simulink model "SPWM_jisuan_simscape"  (R2026a)
settings: Solver=ode23t  StartTime=1  StopTime=2
undefined symbols (not defined in the file): Down, PermanentMagnetSynchrono_class, Up
libraries: fl_lib x12, nesl_utility x10, ee_lib x4, eePwmGenerator x3, eeTransforms x2, elec_conv_HighZElecRef x1
settings Model: Creator=刘炳宏  LastModifiedBy=mushen
settings DebuggingCC: SaveWithParameterizedLinksMsg=none
settings SimscapeCC: SimscapeLogType=none  SimscapeLogDataHistory=5000.0

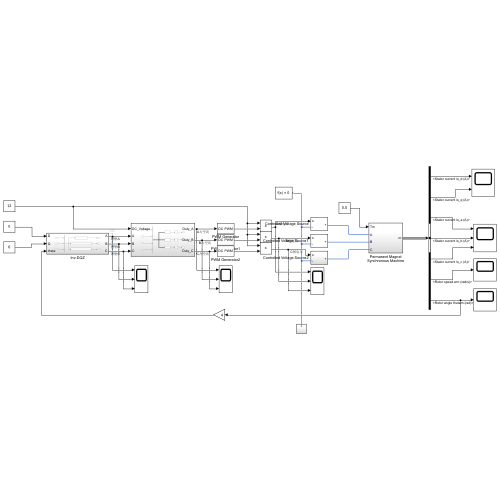
[thumbnail: Simulink's stored preview of the top-level diagram]
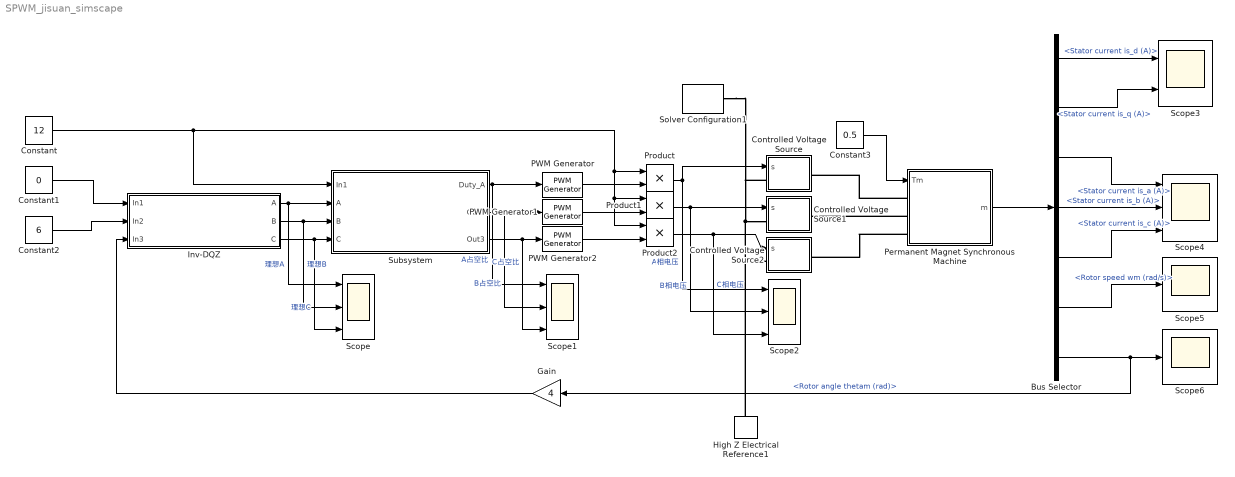
== system SPWM_jisuan_simscape ==
  Bus Selector : BusSelector  OutputSignals=Stator current is_d (A),Stator current is_q (A),Stator current is_a (A),Stator current is_b (A),Stator current is_c (A),Rotor speed wm (rad/s),Rotor angle thetam (rad)
  Constant : Constant  Value=12
  Constant1 : Constant  Value=0
  Constant2 : Constant  Value=6
  Constant3 : Constant  Value=0.5
  Controlled Voltage Source : Subsystem
      settings: OpenFcn=elec.conv.unmask(gcb);
  Controlled Voltage Source1 : Subsystem
      settings: OpenFcn=elec.conv.unmask(gcb);
  Controlled Voltage Source2 : Subsystem
  Gain : Gain  Gain=4
  High Z Electrical Reference1 : elec_conv_HighZElecRef/High Z Electrical Reference  SystemSampleTime=-1  VariantActivationTime=update diagram  EmptyChoice=off  PassThrough=off  PassThroughVariantControl=(default)  EmptyChoiceVariantControl=(default)  AllowFlexibleInterface=on  Latency=0  AutoFrameSizeCalculation=off
  Inv-DQZ : Subsystem
  PWM Generator : eePwmGenerator/PWM Generator  CarrCount=Up-Down  Tper=0.0001  Tdelay=0  Ts=5e-6
  PWM Generator1 : eePwmGenerator/PWM Generator  CarrCount=Up-Down  Tper=0.0001  Tdelay=0  Ts=5e-6
  PWM Generator2 : eePwmGenerator/PWM Generator  CarrCount=Up-Down  Tper=0.0001  Tdelay=0  Ts=5e-6
  Permanent Magnet Synchronous Machine : Subsystem
  Product : Product
  Product1 : Product
  Product2 : Product
  Scope{,1..2,4} (4 alike) : Scope  NumInputPorts=3
      Scope settings: ActiveDisplayYMinimum=-25  ActiveDisplayYMaximum=25
      Scope1 settings: ActiveDisplayYMinimum=-0.12499999999999997  ActiveDisplayYMaximum=1.125
      Scope2 settings: ActiveDisplayYMinimum=-1.5  ActiveDisplayYMaximum=13.5  DataLoggingVariableName=ScopeData2
      Scope4 settings: ActiveDisplayYMinimum=-3.47944  ActiveDisplayYMaximum=3.68146  DataLoggingVariableName=ScopeData4
  Scope3 : Scope  NumInputPorts=2
      settings: ActiveDisplayYMinimum=-3.3984401436548075  ActiveDisplayYMaximum=6.0425246459307287  DataLoggingVariableName=ScopeData3
  Scope5 : Scope
      settings: ActiveDisplayYMinimum=-5.36888  ActiveDisplayYMaximum=42.81454  DataLoggingVariableName=ScopeData5
  Scope6 : Scope
      settings: ActiveDisplayYMinimum=0.00745  ActiveDisplayYMaximum=0.02745  DataLoggingVariableName=ScopeData6
  Solver Configuration1 : nesl_utility/Solver Configuration  PhysicalDomain=network_engine_domain  SubClassName=solver  LeftPortType=input  RightPortType=generic  Tones=[]  Harmonics=[]  SimulateNoise=off  Profile=off  UseLocalSampling=off  EnableSwitchedLinearOptims=on  FrequencyDomain=off  UseCCode=off  RelTol=0.001  AbsTol=0.001  MinStep=1e-09  ToWorkspace=off  RevertToSquareIcSolve=off  NumHomotopyIterations=100  PhasorMode=off  PhasorModeNumHarmonics=1  ConsistencySolver=NEWTON_XTOL_AFTER_FTOL  CanonicalOrdering=CANONICAL  OptimizeIntermediates=OPTIMIZED  IndexReductionMethod=DerivativeReplacement  DoDC=off  ResidualTolerance=1e-09  ConsistencyTolSource=GLOBAL  ConsistencyAbsTol=0.001  ConsistencyRelTol=0.001  ConsistencyTolFactor=0.001  UseLocalSolver=off  LocalSolverChoice=NE_BACKWARD_EULER_ADVANCER  ResolveIndetEquations=on  FunctionEvalNumThread=1  LocalSolverSampleTime=0.001  DoFixedCost=off  MaxNonlinIter=3  MaxModeIter=2  ComputeImpulses=off  ImpulseIterations=2  LinearAlgebra=auto  LinearAlgebraNumThread=0  EquationFormulation=NE_TIME_EF  DelaysMemoryBudget=1024  AutomaticFiltering=on  FilteringTimeConstant=0.001  PartitionStorageMethod=AS_NEEDED  PartitionMemoryBudget=1024  PartitionMethod=ROBUST  MultibodyUseLocalSolver=off  MultibodyLocalSolverChoice=ODE1  MultibodyLocalSolverSampleTime=0.001
  Subsystem : Subsystem
  wires:
  Inv-DQZ/2(B) -> Scope/2, Subsystem/3(B)  "理想B"
  Inv-DQZ/3(C) -> Scope/3, Subsystem/4(C)  "理想C"
  Inv-DQZ/1(A) -> Scope/1, Subsystem/2(A)  "理想A"
  Subsystem/1(Duty_A) -> PWM Generator/1, Scope1/1  "A占空比"
  Subsystem/2(Out2) -> PWM Generator1/1, Scope1/2  "B占空比"
  Subsystem/3(Out3) -> PWM Generator2/1, Scope1/3  "C占空比"
  PWM Generator/1 -> Product/2
  PWM Generator1/1 -> Product1/2
  PWM Generator2/1 -> Product2/2
  Constant/1 -> Product2/1, Product1/1, Product/1, Subsystem/1(In1)
  Constant1/1 -> Inv-DQZ/1(In1)
  Constant2/1 -> Inv-DQZ/2(In2)
  Constant3/1 -> Permanent Magnet Synchronous Machine/1(Tm)
  Product/1 -> Scope2/1, Controlled Voltage Source/1(s)  "A相电压"
  Product1/1 -> Scope2/2, Controlled Voltage Source1/1(s)  "B相电压"
  Product2/1 -> Scope2/3, Controlled Voltage Source2/1(s)  "C相电压"
  Permanent Magnet Synchronous Machine/1(m) -> Bus Selector/1
  Bus Selector/1 -> Scope3/1  "<Stator current is_d (A)>"
  Bus Selector/2 -> Scope3/2  "<Stator current is_q (A)>"
  Bus Selector/4 -> Scope4/2  "<Stator current is_b (A)>"
  Bus Selector/3 -> Scope4/1  "<Stator current is_a (A)>"
  Bus Selector/5 -> Scope4/3  "<Stator current is_c (A)>"
  Bus Selector/6 -> Scope5/1  "<Rotor speed wm (rad/s)>"
  Bus Selector/7 -> Gain/1, Scope6/1  "<Rotor angle thetam (rad)>"
  Gain/1 -> Inv-DQZ/3(In3)
  connections:
  Permanent Magnet Synchronous Machine/LConn2 -- Controlled Voltage Source1/RConn1
  Permanent Magnet Synchronous Machine/LConn3 -- Controlled Voltage Source2/RConn1
  Permanent Magnet Synchronous Machine/LConn1 -- Controlled Voltage Source/RConn1
  Controlled Voltage Source/LConn1 -- Solver Configuration1/RConn1 -- Controlled Voltage Source1/LConn1 -- Controlled Voltage Source2/LConn1 -- High Z Electrical Reference1/LConn1

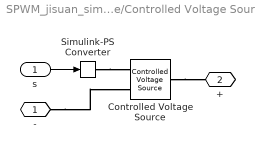
== system SPWM_jisuan_simscape/Controlled Voltage Source ==
  s : Inport
  Controlled Voltage Source : fl_lib/Electrical/Electrical Sources/Controlled Voltage Source
  Simulink-PS Converter : nesl_utility/Simulink-PS Converter  PhysicalDomain=network_engine_domain  SubClassName=ps_input  LeftPortType=input  RightPortType=output  PseudoPeriodic=off  Frequencies=[]  NoiseDistribution=none  NoiseParameters=[]  Unit=1  AffineConversion=off  FilteringAndDerivatives=provide  SimscapeFilterOrder=1  InputFilterTimeConstant=0.001  UdotUserProvided=0
  - : PMIOPort  Side=Left
  + : PMIOPort  Port=2  Side=Right
  wires:
  s/1 -> Simulink-PS Converter/1
  connections:
  -/RConn1 -- Controlled Voltage Source/RConn2
  Simulink-PS Converter/RConn1 -- Controlled Voltage Source/RConn1
  Controlled Voltage Source/LConn1 -- +/RConn1

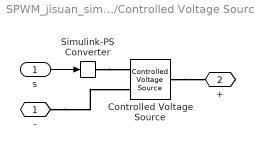
== system SPWM_jisuan_simscape/Controlled Voltage Source1 ==
  s : Inport
  Controlled Voltage Source : fl_lib/Electrical/Electrical Sources/Controlled Voltage Source
  Simulink-PS Converter : nesl_utility/Simulink-PS Converter  PhysicalDomain=network_engine_domain  SubClassName=ps_input  LeftPortType=input  RightPortType=output  PseudoPeriodic=off  Frequencies=[]  NoiseDistribution=none  NoiseParameters=[]  Unit=1  AffineConversion=off  FilteringAndDerivatives=provide  SimscapeFilterOrder=1  InputFilterTimeConstant=0.001  UdotUserProvided=0
  - : PMIOPort  Side=Left
  + : PMIOPort  Port=2  Side=Right
  wires:
  s/1 -> Simulink-PS Converter/1
  connections:
  -/RConn1 -- Controlled Voltage Source/RConn2
  Simulink-PS Converter/RConn1 -- Controlled Voltage Source/RConn1
  Controlled Voltage Source/LConn1 -- +/RConn1

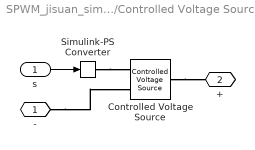
== system SPWM_jisuan_simscape/Controlled Voltage Source2 ==
  s : Inport
  Controlled Voltage Source : fl_lib/Electrical/Electrical Sources/Controlled Voltage Source
  Simulink-PS Converter : nesl_utility/Simulink-PS Converter  PhysicalDomain=network_engine_domain  SubClassName=ps_input  LeftPortType=input  RightPortType=output  PseudoPeriodic=off  Frequencies=[]  NoiseDistribution=none  NoiseParameters=[]  Unit=1  AffineConversion=off  FilteringAndDerivatives=provide  SimscapeFilterOrder=1  InputFilterTimeConstant=0.001  UdotUserProvided=0
  - : PMIOPort  Side=Left
  + : PMIOPort  Port=2  Side=Right
  wires:
  s/1 -> Simulink-PS Converter/1
  connections:
  -/RConn1 -- Controlled Voltage Source/RConn2
  Simulink-PS Converter/RConn1 -- Controlled Voltage Source/RConn1
  Controlled Voltage Source/LConn1 -- +/RConn1

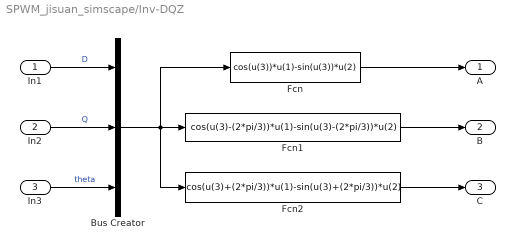
== system SPWM_jisuan_simscape/Inv-DQZ ==
  In1 : Inport
  In2 : Inport  Port=2
  In3 : Inport  Port=3
  Bus Creator : BusCreator  Inputs=3
  Fcn : Fcn  Expr=cos(u(3))*u(1)-sin(u(3))*u(2)
  Fcn1 : Fcn  Expr=cos(u(3)-(2*pi/3))*u(1)-sin(u(3)-(2*pi/3))*u(2)
  Fcn2 : Fcn  Expr=cos(u(3)+(2*pi/3))*u(1)-sin(u(3)+(2*pi/3))*u(2)
  A : Outport
  B : Outport  Port=2
  C : Outport  Port=3
  wires:
  In3/1 -> Bus Creator/3  "theta"
  In2/1 -> Bus Creator/2  "Q"
  In1/1 -> Bus Creator/1  "D"
  Bus Creator/1 -> Fcn/1, Fcn1/1, Fcn2/1
  Fcn/1 -> A/1
  Fcn1/1 -> B/1
  Fcn2/1 -> C/1

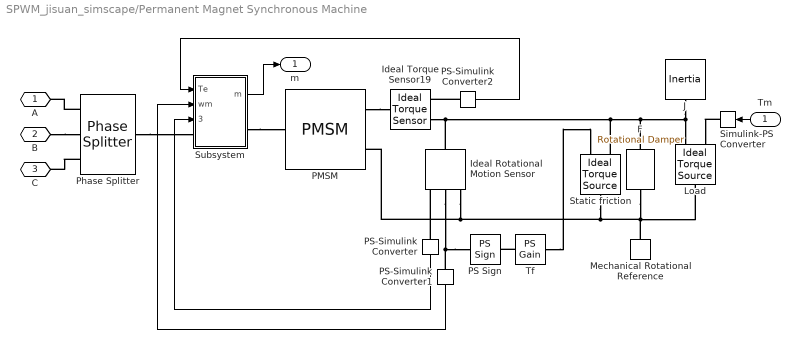
== system SPWM_jisuan_simscape/Permanent Magnet Synchronous Machine ==
  Tm : Inport
  F : fl_lib/Mechanical/Rotational Elements/Rotational Damper  D=0.0003505 N*m/(rad/s)  w_specify=on  w_priority=High  w=0 rad/s  w_nominal_specify=off  w_nominal_value=1  w_nominal_unit=rad/s  t_specify=off  t_priority=None  t=0 N*m  t_nominal_specify=off  t_nominal_value=1  t_nominal_unit=N*m
  Ideal Rotational Motion Sensor : fl_lib/Mechanical/Mechanical Sensors/Ideal Rotational Motion Sensor  reference=foundation.enum.MeasurementReference.difference  acceleration_port=false  velocity_port=true  position_port=true  wrap_angle=simscape.enum.onoff.off  offset=1 deg
  Ideal Torque Sensor19 : fl_lib/Mechanical/Mechanical Sensors/Ideal Torque Sensor
  J : fl_lib/Mechanical/Rotational Elements/Inertia  inertia=0.00062 kg*m^2  num_ports=foundation.enum.numPorts2.one  w_specify=on  w_priority=High  w=0 rad/s  w_nominal_specify=off  w_nominal_value=1  w_nominal_unit=rad/s  t_specify=off  t_priority=None  t=0 N*m  t_nominal_specify=off  t_nominal_value=1  t_nominal_unit=N*m
  Load : fl_lib/Mechanical/Mechanical Sources/Ideal Torque Source
  Mechanical Rotational Reference : fl_lib/Mechanical/Rotational Elements/Mechanical Rotational Reference
  PMSM : ee_lib/Electromechanical/Permanent Magnet/PMSM  port_option=ee.enum.threePhasePort.composite  winding_type=ee.enum.statorconnection.wye  machine_param=ee.enum.pmsm.parameterization.constant  nPolePairs=4  pmflux_param=1  pm_flux_linkage=PermanentMagnetSynchrono_class('Torque Tm',[0.00062 0.0003505 4 0],4,'Flux linkage established by magnets (V.s)',0.074147,53.7951,0.44488,'Aligned with phase A axis (original Park)',[0 1 0 0],'Sinusoidal',120,'3',[0 0 0 0 0 0]).objParamMappingDerived.NewDerivedParam.pm_flux_linkage Wb  torque_constant=0.18 N*m/A  back_emf_constant=0.18 V/(rad/s)  stator_param=1  Ld=0.0085 H  Lq=0.0085 H  idVec=[-200, 0, 200] A  iqVec=[-200, 0, 200] A  LdMatrix=0.0002 * ones(3, 3) H  LqMatrix=0.0002 * ones(3, 3) H  PmMatrix=0.1 * ones(3, 3) Wb  ktMatrix=0.18 * ones(3, 3) N*m/A  keMatrix=0.18 * ones(3, 3) V/(rad/s)  L0=1e-09 H  Ls=0.0002 H  Lm=-0.00002 H  Ms=0.00002 H  Rs=0.18 Ohm  zero_sequence=0  axes_param=2  loss_param=ee.enum.ironloss.none  losses_oc=[0, 0, 0] W  losses_sc=[0, 0, 0] W  f_losses=60 Hz  Isc_losses=95 A  J=0 kg*m^2  lam=0 N*m/(rad/s)  i_d_specify=on  i_d_priority=High  i_d=PermanentMagnetSynchrono_class('Torque Tm',[0.00062 0.0003505 4 0],4,'Flux linkage established by magnets (V.s)',0.074147,53.7951,0.44488,'Aligned with phase A axis (original Park)',[0 1 0 0],'Sinusoidal',120,'3',[0 0 0 0 0 0]).objParamMappingDerived.NewDerivedParam.i_d A  i_d_nominal_specify=off  i_d_nominal_value=1  i_d_nominal_unit=A  i_q_specify=on  i_q_priority=High  i_q=PermanentMagnetSynchrono_class('Torque Tm',[0.00062 0.0003505 4 0],4,'Flux linkage established by magnets (V.s)',0.074147,53.7951,0.44488,'Aligned with phase A axis (original Park)',[0 1 0 0],'Sinusoidal',120,'3',[0 0 0 0 0 0]).objParamMappingDerived.NewDerivedParam.i_q A  i_q_nominal_specify=off  i_q_nominal_value=1  i_q_nominal_unit=A  torque_specify=off  torque_priority=None  torque=0 N*m  torque_nominal_specify=off  torque_nominal_value=1  torque_nominal_unit=N*m  angular_velocity_specify=on  angular_velocity_priority=High  angular_velocity=0 rad/s  angular_velocity_nominal_specify=off  angular_velocity_nominal_value=1  angular_velocity_nominal_unit=rpm  angular_position_specify=on  angular_position_priority=High  angular_position=1 deg  angular_position_nominal_specify=off  angular_position_nominal_value=1  angular_position_nominal_unit=deg  alpha=3.93e-3 1/K  alpha_flux=-0.001 1/K  Tmeas=298.15 K  stator_thermal_mass=100 J/K  rotor_thermal_mass=200 J/K  Rm_percent_rotor=90  Rd_percent_rotor=30  temperatureA_specify=off  temperatureA_priority=High  temperatureA=25 degC  temperatureA_nominal_specify=off  temperatureA_nominal_value=1  temperatureA_nominal_unit=degC  temperatureB_specify=off  temperatureB_priority=High  temperatureB=25 degC  temperatureB_nominal_specify=off  temperatureB_nominal_value=1  temperatureB_nominal_unit=degC  temperatureC_specify=off  temperatureC_priority=High  temperatureC=25 degC  temperatureC_nominal_specify=off  temperatureC_nominal_value=1  temperatureC_nominal_unit=degC  temperatureR_specify=off  temperatureR_priority=High  temperatureR=25 degC  temperatureR_nominal_specify=off  temperatureR_nominal_value=1  temperatureR_nominal_unit=degC
  PS Sign : fl_lib/Physical Signals/Nonlinear Operators/PS Sign
  PS-Simulink Converter : nesl_utility/PS-Simulink Converter  PhysicalDomain=network_engine_domain  SubClassName=ps_output  LeftPortType=input  RightPortType=output  PseudoPeriodic=off  Frequencies=[]  VectorFormat=1-D array  Unit=1  AffineConversion=off
  PS-Simulink Converter1 : nesl_utility/PS-Simulink Converter  PhysicalDomain=network_engine_domain  SubClassName=ps_output  LeftPortType=input  RightPortType=output  PseudoPeriodic=off  Frequencies=[]  VectorFormat=1-D array  Unit=1  AffineConversion=off
  PS-Simulink Converter2 : nesl_utility/PS-Simulink Converter  PhysicalDomain=network_engine_domain  SubClassName=ps_output  LeftPortType=input  RightPortType=output  PseudoPeriodic=off  Frequencies=[]  VectorFormat=1-D array  Unit=1  AffineConversion=off
  Phase Splitter : ee_lib/Connectors & References/Phase Splitter
  Simulink-PS Converter : nesl_utility/Simulink-PS Converter  PhysicalDomain=network_engine_domain  SubClassName=ps_input  LeftPortType=input  RightPortType=output  PseudoPeriodic=off  Frequencies=[]  NoiseDistribution=none  NoiseParameters=[]  Unit=1  AffineConversion=off  FilteringAndDerivatives=provide  SimscapeFilterOrder=1  InputFilterTimeConstant=0.001  UdotUserProvided=0
  Static friction : fl_lib/Mechanical/Mechanical Sources/Ideal Torque Source
  Subsystem : Subsystem
  Tf : fl_lib/Physical Signals/Functions/PS Gain  gain=PermanentMagnetSynchrono_class('Torque Tm',[0.00062 0.0003505 4 0],4,'Flux linkage established by magnets (V.s)',0.074147,53.7951,0.44488,'Aligned with phase A axis (original Park)',[0 1 0 0],'Sinusoidal',120,'3',[0 0 0 0 0 0]).objParamMappingDerived.NewDerivedParam.Tf
  A : PMIOPort  Side=Left
  B : PMIOPort  Port=2  Side=Left
  C : PMIOPort  Port=3  Side=Left
  m : Outport  VectorParamsAs1DForOutWhenUnconnected=off
  wires:
  PS-Simulink Converter1/1 -> Subsystem/2(wm)
  PS-Simulink Converter/1 -> Subsystem/3(thetam)
  PS-Simulink Converter2/1 -> Subsystem/1(Te)
  Subsystem/1(m) -> m/1
  Tm/1 -> Simulink-PS Converter/1
  connections:
  PS-Simulink Converter2/LConn1 -- Ideal Torque Sensor19/RConn2
  Phase Splitter/LConn1 -- Subsystem/LConn1
  Subsystem/RConn1 -- PMSM/LConn1
  PS-Simulink Converter/LConn1 -- Ideal Rotational Motion Sensor/RConn3
  Tf/RConn1 -- Static friction/RConn1
  PS Sign/LConn1 -- PS-Simulink Converter1/LConn1 -- Ideal Rotational Motion Sensor/RConn2
  Tf/LConn1 -- PS Sign/RConn1
  PMSM/RConn1 -- Ideal Torque Sensor19/LConn1
  Ideal Torque Sensor19/RConn1 -- Static friction/RConn2 -- F/LConn1 -- Load/RConn2 -- J/LConn1 -- Ideal Rotational Motion Sensor/LConn1
  Phase Splitter/RConn3 -- C/RConn1
  Phase Splitter/RConn1 -- A/RConn1
  B/RConn1 -- Phase Splitter/RConn2
  Simulink-PS Converter/RConn1 -- Load/RConn1
  Load/LConn1 -- F/RConn1 -- Static friction/LConn1 -- PMSM/RConn2 -- Ideal Rotational Motion Sensor/RConn1 -- Mechanical Rotational Reference/LConn1

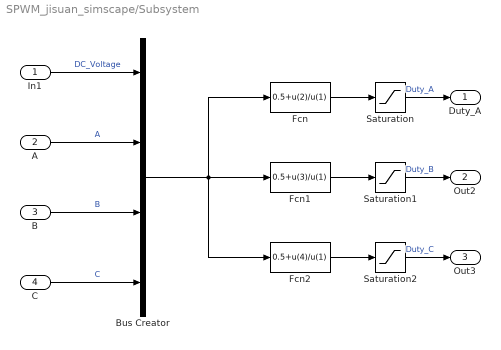
== system SPWM_jisuan_simscape/Subsystem ==
  In1 : Inport
  A : Inport  Port=2
  B : Inport  Port=3
  C : Inport  Port=4
  Bus Creator : BusCreator  Inputs=4
  Fcn : Fcn  Expr=0.5+u(2)/u(1)
  Fcn1 : Fcn  Expr=0.5+u(3)/u(1)
  Fcn2 : Fcn  Expr=0.5+u(4)/u(1)
  Saturation : Saturate  UpperLimit=1  LowerLimit=0
  Saturation1 : Saturate  UpperLimit=1  LowerLimit=0
  Saturation2 : Saturate  UpperLimit=1  LowerLimit=0
  Duty_A : Outport
  Out2 : Outport  Port=2
  Out3 : Outport  Port=3
  wires:
  In1/1 -> Bus Creator/1  "DC_Voltage"
  A/1 -> Bus Creator/2  "A"
  B/1 -> Bus Creator/3  "B"
  C/1 -> Bus Creator/4  "C"
  Fcn/1 -> Saturation/1
  Bus Creator/1 -> Fcn/1, Fcn2/1, Fcn1/1
  Saturation/1 -> Duty_A/1  "Duty_A"
  Saturation1/1 -> Out2/1  "Duty_B"
  Fcn1/1 -> Saturation1/1
  Saturation2/1 -> Out3/1  "Duty_C"
  Fcn2/1 -> Saturation2/1

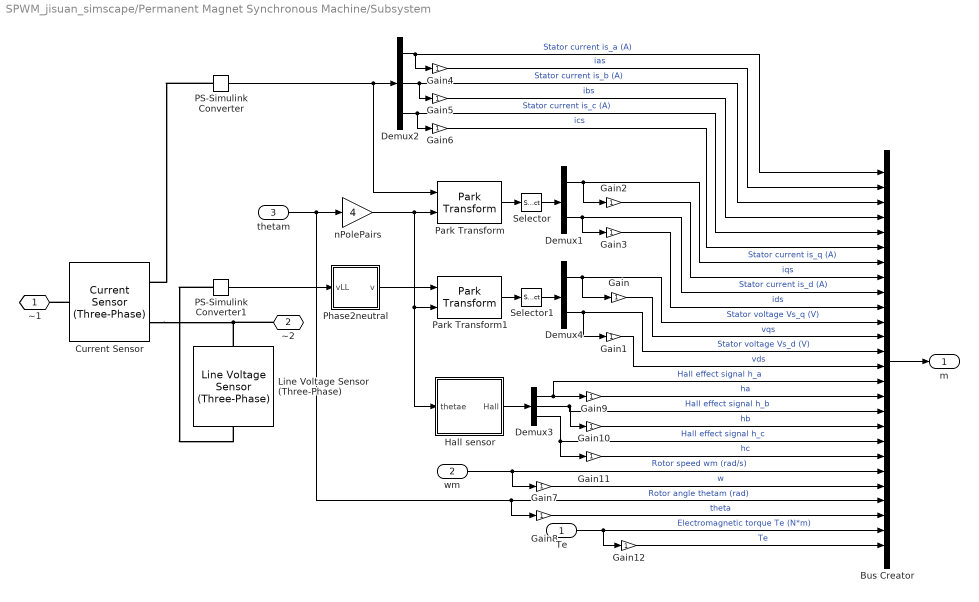
== system SPWM_jisuan_simscape/Permanent Magnet Synchronous Machine/Subsystem ==
  Te : Inport
  wm : Inport  Port=2
  thetam : Inport  Port=3
  Bus Creator : BusCreator  Inputs=26
  Current Sensor : ee_lib/Sensors & Transducers/Current Sensor (Three-Phase)  port_option=ee.enum.threePhasePort.composite
  Demux1 : Demux  Outputs=2
  Demux2 : Demux  Outputs=3
  Demux3 : Demux  Outputs=3
  Demux4 : Demux  Outputs=2
  Gain{,1..12} (13 alike) : Gain
  Hall sensor : Subsystem
  Line Voltage Sensor (Three-Phase) : ee_lib/Sensors & Transducers/Line Voltage Sensor (Three-Phase)  port_option=ee.enum.threePhasePort.composite
  PS-Simulink Converter : nesl_utility/PS-Simulink Converter  PhysicalDomain=network_engine_domain  SubClassName=ps_output  LeftPortType=input  RightPortType=output  PseudoPeriodic=off  Frequencies=[]  VectorFormat=1-D array  Unit=1  AffineConversion=off
  PS-Simulink Converter1 : nesl_utility/PS-Simulink Converter  PhysicalDomain=network_engine_domain  SubClassName=ps_output  LeftPortType=input  RightPortType=output  PseudoPeriodic=off  Frequencies=[]  VectorFormat=1-D array  Unit=1  AffineConversion=off
  Park Transform : eeTransforms/Park Transform  AxisAlignment=D-axis  PowerInvariant=off
  Park Transform1 : eeTransforms/Park Transform  AxisAlignment=D-axis  PowerInvariant=off
  Phase2neutral : Subsystem
  Selector : Selector  InputPortWidth=3  IndexOptions=Index vector (dialog)  Indices=[2 1]  OutputSizes=1
  Selector1 : Selector  InputPortWidth=3  IndexOptions=Index vector (dialog)  Indices=[2 1]  OutputSizes=1
  nPolePairs : Gain  Gain=4
  ~1 : PMIOPort  Side=Left
  ~2 : PMIOPort  Port=2  Side=Right
  m : Outport  VectorParamsAs1DForOutWhenUnconnected=off
  wires:
  Phase2neutral/1(v) -> Park Transform1/1
  Gain8/1 -> Bus Creator/24  "theta"
  Gain7/1 -> Bus Creator/22  "w"
  Selector1/1 -> Demux4/1
  Selector/1 -> Demux1/1
  Gain11/1 -> Bus Creator/20  "hc"
  Gain10/1 -> Bus Creator/18  "hb"
  Gain9/1 -> Bus Creator/16  "ha"
  Gain1/1 -> Bus Creator/14  "vds"
  Gain/1 -> Bus Creator/12  "vqs"
  Gain3/1 -> Bus Creator/10  "ids"
  Gain2/1 -> Bus Creator/8  "iqs"
  Hall sensor/1(Hall) -> Demux3/1
  PS-Simulink Converter1/1 -> Phase2neutral/1(vLL)
  Gain6/1 -> Bus Creator/6  "ics"
  Gain5/1 -> Bus Creator/4  "ibs"
  Gain4/1 -> Bus Creator/2  "ias"
  PS-Simulink Converter/1 -> Demux2/1, Park Transform/1
  Te/1 -> Bus Creator/25, Gain12/1  "Electromagnetic torque Te (N*m)"
  Gain12/1 -> Bus Creator/26  "Te"
  Demux3/3 -> Bus Creator/19, Gain11/1  "Hall effect signal h_c"
  Demux3/2 -> Gain10/1, Bus Creator/17  "Hall effect signal h_b"
  Demux3/1 -> Gain9/1, Bus Creator/15  "Hall effect signal h_a"
  thetam/1 -> nPolePairs/1, Gain8/1, Bus Creator/23  "Rotor angle thetam (rad)"
  Bus Creator/1 -> m/1
  Demux2/3 -> Bus Creator/5, Gain6/1  "Stator current is_c (A)"
  Demux2/2 -> Gain5/1, Bus Creator/3  "Stator current is_b (A)"
  Demux2/1 -> Gain4/1, Bus Creator/1  "Stator current is_a (A)"
  Demux1/2 -> Gain3/1, Bus Creator/9  "Stator current is_d (A)"
  Park Transform/1 -> Selector/1
  Demux1/1 -> Gain2/1, Bus Creator/7  "Stator current is_q (A)"
  Demux4/2 -> Gain1/1, Bus Creator/13  "Stator voltage Vs_d (V)"
  Demux4/1 -> Gain/1, Bus Creator/11  "Stator voltage Vs_q (V)"
  Park Transform1/1 -> Selector1/1
  nPolePairs/1 -> Hall sensor/1(thetae), Park Transform1/2, Park Transform/2
  wm/1 -> Bus Creator/21, Gain7/1  "Rotor speed wm (rad/s)"
  connections:
  PS-Simulink Converter1/LConn1 -- Line Voltage Sensor (Three-Phase)/RConn1
  PS-Simulink Converter/LConn1 -- Current Sensor/RConn1
  ~2/RConn1 -- Line Voltage Sensor (Three-Phase)/LConn1 -- Current Sensor/RConn2
  Current Sensor/LConn1 -- ~1/RConn1

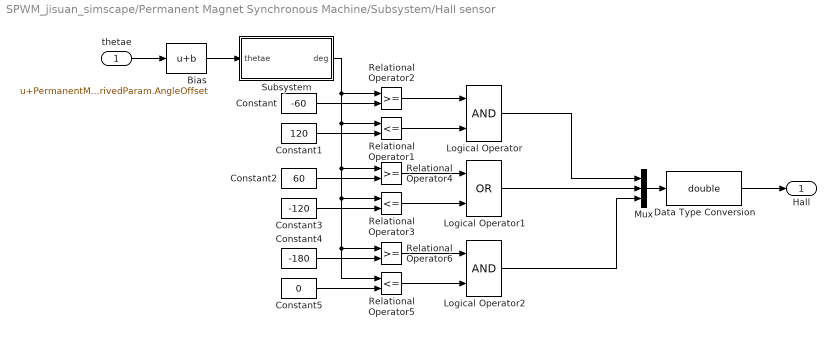
== system SPWM_jisuan_simscape/Permanent Magnet Synchronous Machine/Subsystem/Hall sensor ==
  thetae : Inport
  Bias : Bias  Bias=PermanentMagnetSynchrono_class('Torque Tm',[0.00062 0.0003505 4 0],4,'Flux linkage established by magnets (V.s)',0.074147,53.7951,0.44488,'Aligned with phase A axis (original Park)',[0 1 0 0],'Sinusoidal',120,'3',[0 0 0 0 0 0]).objParamMappingDerived.NewDerivedParam.AngleOffset  SaturateOnIntegerOverflow=off
  Constant : Constant  Value=-60
  Constant1 : Constant  Value=120
  Constant2 : Constant  Value=60
  Constant3 : Constant  Value=-120
  Constant4 : Constant  Value=-180
  Constant5 : Constant  Value=0
  Data Type Conversion : DataTypeConversion  OutDataTypeStr=double  SaturateOnIntegerOverflow=off  RndMeth=Floor
  Logical Operator : Logic  AllPortsSameDT=off  OutDataTypeStr=boolean
  Logical Operator1 : Logic  Operator=OR  AllPortsSameDT=off  OutDataTypeStr=boolean
  Logical Operator2 : Logic  AllPortsSameDT=off  OutDataTypeStr=boolean
  Mux : Mux  Inputs=3
  Relational Operator1 : RelationalOperator  Operator=<=
  Relational Operator2 : RelationalOperator
  Relational Operator3 : RelationalOperator  Operator=<=
  Relational Operator4 : RelationalOperator
  Relational Operator5 : RelationalOperator  Operator=<=
  Relational Operator6 : RelationalOperator
  Subsystem : Subsystem
  Hall : Outport  VectorParamsAs1DForOutWhenUnconnected=off
  wires:
  Bias/1 -> Subsystem/1(thetae)
  Data Type Conversion/1 -> Hall/1
  thetae/1 -> Bias/1
  Constant2/1 -> Relational Operator4/2
  Constant1/1 -> Relational Operator1/2
  Relational Operator4/1 -> Logical Operator1/1
  Constant/1 -> Relational Operator2/2
  Subsystem/1(deg) -> Relational Operator2/1, Relational Operator1/1, Relational Operator6/1, Relational Operator5/1, Relational Operator3/1, Relational Operator4/1
  Relational Operator1/1 -> Logical Operator/2
  Relational Operator2/1 -> Logical Operator/1
  Mux/1 -> Data Type Conversion/1
  Relational Operator3/1 -> Logical Operator1/2
  Constant5/1 -> Relational Operator5/2
  Constant4/1 -> Relational Operator6/2
  Relational Operator6/1 -> Logical Operator2/1
  Relational Operator5/1 -> Logical Operator2/2
  Logical Operator/1 -> Mux/1
  Logical Operator1/1 -> Mux/2
  Logical Operator2/1 -> Mux/3
  Constant3/1 -> Relational Operator3/2

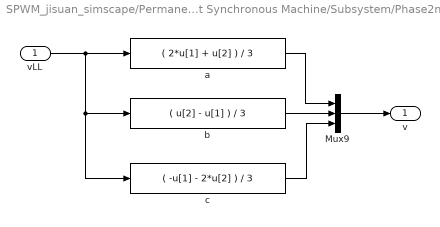
== system SPWM_jisuan_simscape/Permanent Magnet Synchronous Machine/Subsystem/Phase2neutral ==
  vLL : Inport
  Mux9 : Mux  Inputs=3
  a : Fcn  Expr=( 2*u[1] + u[2] ) / 3
  b : Fcn  Expr=( u[2] - u[1] ) / 3
  c : Fcn  Expr=( -u[1] - 2*u[2] ) / 3
  v : Outport
  wires:
  b/1 -> Mux9/2
  vLL/1 -> b/1, c/1, a/1
  c/1 -> Mux9/3
  a/1 -> Mux9/1
  Mux9/1 -> v/1

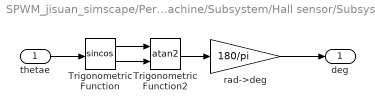
== system SPWM_jisuan_simscape/Permanent Magnet Synchronous Machine/Subsystem/Hall sensor/Subsystem ==
  thetae : Inport
  Trigonometric Function : Trigonometry  Operator=sincos
  Trigonometric Function2 : Trigonometry  Operator=atan2
  rad->deg : Gain  Gain=180/pi  SaturateOnIntegerOverflow=on  OutDataTypeStr=Inherit: Same as input  ParamDataTypeStr=Inherit: Same as input
  deg : Outport  VectorParamsAs1DForOutWhenUnconnected=off
  wires:
  thetae/1 -> Trigonometric Function/1
  Trigonometric Function/2 -> Trigonometric Function2/2
  rad->deg/1 -> deg/1
  Trigonometric Function/1 -> Trigonometric Function2/1
  Trigonometric Function2/1 -> rad->deg/1
